simulink model "inverter_single_phase_off_grid"  (R2024a)
settings: Solver=FixedStepAuto  StartTime=0.0  StopTime=2  MaxStep=1e-7  MinStep=1e-8  RelTol=1e-3
libraries: spsMosfetLib x4, spsSeriesRLCBranchLib x4, spsCurrentMeasurementLib x2, spsVoltageMeasurementLib x2, spsDCVoltageSourceLib x1, spsTriangleGeneratorLib x1, sps_lib x1
settings Model: PacingRate=100000  Creator=Administrator  LastModifiedBy=50803

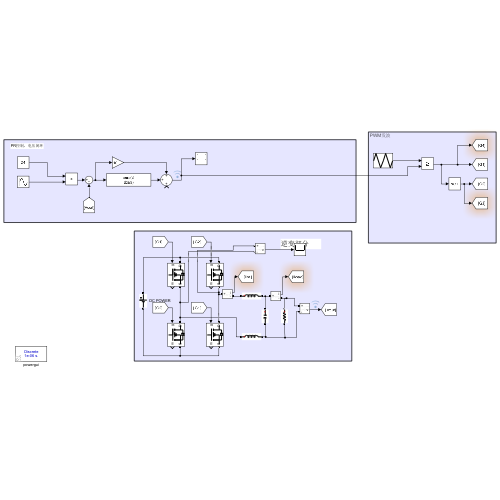
[thumbnail: Simulink's stored preview of the top-level diagram]
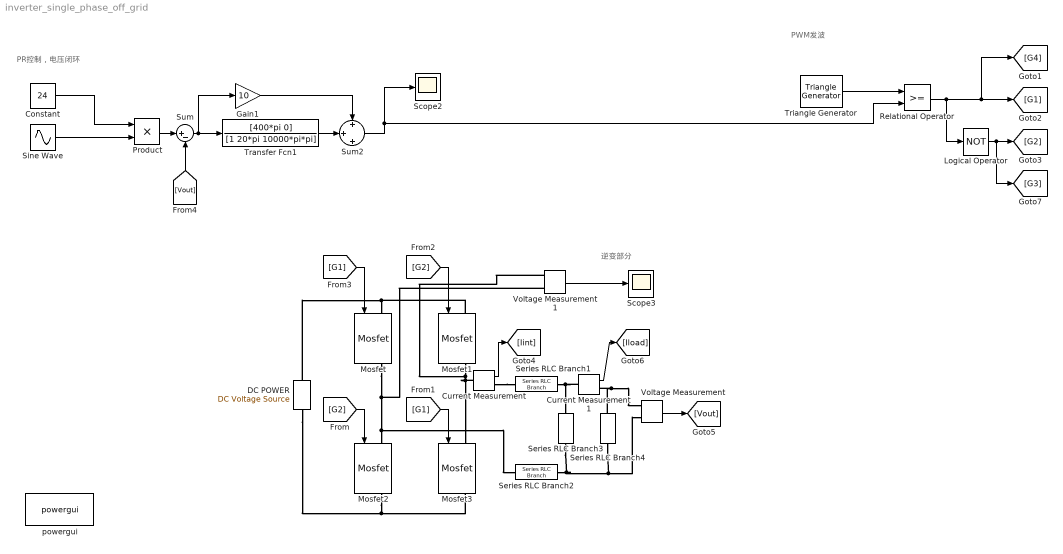
== system inverter_single_phase_off_grid ==
  note: PR控制，电压闭环
  note: PWM发波
  note: 逆变部分
  Constant : Constant  Value=24
  Current Measurement : spsCurrentMeasurementLib/Current Measurement  PhasorSimulation=off  OutputType=Complex  PSBequivalent=0
  Current Measurement1 : spsCurrentMeasurementLib/Current Measurement  PhasorSimulation=off  OutputType=Complex  PSBequivalent=0
  DC POWER : spsDCVoltageSourceLib/DC Voltage Source  Amplitude=48  Measurements=None
  Gain1 : Gain  Gain=10
  Logical Operator : Logic  Operator=NOT  AllPortsSameDT=off  OutDataTypeStr=boolean
  Mosfet{,1..3} (4 alike) : spsMosfetLib/Mosfet  Ron=0.1  Lon=0  Rd=0.01  Vfd=0  IC=0  Rs=1e5  Cs=inf  Measurements=on
  Product : Product
  Relational Operator : RelationalOperator  OutDataTypeStr=boolean  RndMeth=Simplest  InputSameDT=off
  Scope2 : Scope
  Scope3 : Scope
  Series RLC Branch1 : spsSeriesRLCBranchLib/Series RLC Branch  LConnTagsString=__new0  RConnTagsString=__new0  BranchType=L  Resistance=0.01  Inductance=5*1e-3  SetiL0=off  InitialCurrent=0  Capacitance=0  Setx0=off  InitialVoltage=0  Measurements=None
  Series RLC Branch2 : spsSeriesRLCBranchLib/Series RLC Branch  LConnTagsString=__new0  RConnTagsString=__new0  BranchType=L  Resistance=0.01  Inductance=5*1e-3  SetiL0=off  InitialCurrent=0  Capacitance=0  Setx0=off  InitialVoltage=0  Measurements=None
  Series RLC Branch3 : spsSeriesRLCBranchLib/Series RLC Branch  LConnTagsString=__new0  RConnTagsString=__new0  BranchType=C  Resistance=0.01  Inductance=1e-3  SetiL0=off  InitialCurrent=0  Capacitance=50*1e-6  Setx0=off  InitialVoltage=0  Measurements=None
  Series RLC Branch4 : spsSeriesRLCBranchLib/Series RLC Branch  LConnTagsString=__new0  RConnTagsString=__new0  BranchType=R  Resistance=6  Inductance=1e-3  SetiL0=off  InitialCurrent=0  Capacitance=182.6*1e-3  Setx0=off  InitialVoltage=0  Measurements=None
  Sine Wave : Sin  Frequency=100*pi  SampleTime=0
  Sum : Sum  Inputs=|+-
  Sum2 : Sum  Inputs=+|+|+
  Transfer Fcn1 : TransferFcn  Numerator=[400*pi 0]  Denominator=[1 20*pi 10000*pi*pi]
  Triangle Generator : spsTriangleGeneratorLib/Triangle Generator  Freq=1e4  Phase=90  Ts=0
  Voltage Measurement : spsVoltageMeasurementLib/Voltage Measurement  PhasorSimulation=off  OutputType=Complex  PSBequivalent=0
  Voltage Measurement1 : spsVoltageMeasurementLib/Voltage Measurement  PhasorSimulation=off  OutputType=Complex  PSBequivalent=0
  powergui : sps_lib/powergui  Priority=1  SimulationMode=Discrete  SampleTime=1e-6  frequency=60  Iterations=50  frequencyindice=0  Pbase=100e6  ErrMax=1e-4  UnitsV=kV  UnitsW=MW  buscounter=0  FunctionMessages=off  echomessages=off  EnableUseOfTLC=off  CurrentSourceSwitches=off  DisableSnubberDevices=off  DisableRonSwitches=off  DisableVfSwitches=off  DisplayEquations=off  AutomaticDiscreteSolvers=off  SolverType=Tustin/Backward Euler (TBE)  Interpol=off  ExternalGateDelay=off  methode=off  Ts=100  x0status=blocks  SPID=on  SwTol=0  HookPort=off  NonlinearTolerance=1e-4  nMaxIteration=100  ContinueOnMaxIteration=off  RestoreLinks=warning  ResistiveCurrentMeasurement=off  Frange=[0:2:500]  Ylog=off  Xlog=on  ShowGrid=off  save=off  variable=ZData  structure=0  ZoomFFT=off  StartTime=0.0  cycles=1  DisplayStyle=1  fundamental=60  FreqAxis=off  MaxFrequency=1000  frequencyindicesteady=1  RmsSteady=1  display=off
  wires:
  [G1] -> Mosfet/1
  [G2] -> Mosfet1/1
  [G1] -> Mosfet3/1
  [G2] -> Mosfet2/1
  Current Measurement/1 -> [Iint]
  Current Measurement1/1 -> [Iload]
  [Vout] -> Sum/2
  Sum/1 -> Transfer Fcn1/1, Gain1/1
  Transfer Fcn1/1 -> Sum2/2
  Gain1/1 -> Sum2/1
  Sum2/1 -> Relational Operator/2, Scope2/1
  Triangle Generator/1 -> Relational Operator/1
  Relational Operator/1 -> [G4], [G1], Logical Operator/1
  Logical Operator/1 -> [G3], [G2]
  Constant/1 -> Product/1
  Sine Wave/1 -> Product/2
  Product/1 -> Sum/1
  Voltage Measurement1/1 -> Scope3/1
  Voltage Measurement/1 -> [Vout]
  connections:
  Mosfet/LConn1 -- DC POWER/RConn1 -- Mosfet1/LConn1
  Mosfet1/RConn1 -- Voltage Measurement1/LConn1 -- Current Measurement/LConn1 -- Mosfet3/LConn1
  Mosfet3/RConn1 -- DC POWER/LConn1 -- Mosfet2/RConn1
  Mosfet2/LConn1 -- Voltage Measurement1/LConn2 -- Mosfet/RConn1 -- Series RLC Branch2/LConn1
  Series RLC Branch1/RConn1 -- Current Measurement1/LConn1 -- Series RLC Branch3/LConn1
  Current Measurement/RConn1 -- Series RLC Branch1/LConn1
  Series RLC Branch4/LConn1 -- Voltage Measurement/LConn1 -- Current Measurement1/RConn1
  Series RLC Branch2/RConn1 -- Series RLC Branch4/RConn1 -- Voltage Measurement/LConn2 -- Series RLC Branch3/RConn1
